simulink model "Schema_inteco_2"  (R2022b)
settings: Solver=VariableStepAuto  StartTime=0.0  StopTime=60  RelTol=1e-3
undefined symbols (not defined in the file): fm, g, Jm, Jphi, kb, kl, L, m, M, R, Ts, w
settings Model: Creator=Bogdana Cazan  LastModifiedBy=georg
settings SolverCC: AlgebraicLoopSolver=TrustRegion
settings DataIOCC: ReturnWorkspaceOutputs=off
settings DebuggingCC: UnconnectedInputMsg=warning  UnconnectedOutputMsg=warning  UnconnectedLineMsg=warning  SFMachineParentedDataDiag=warning  ArithmeticOperatorsInVariantConditions=warning
settings ModelReferenceCC: EnableRefExpFcnMdlSchedulingChecks=on
settings SFSimCC: CustomCodeUndefinedFunction=UseInterfaceOnly
settings RTWCC: DLArmComputeVersion=19.05

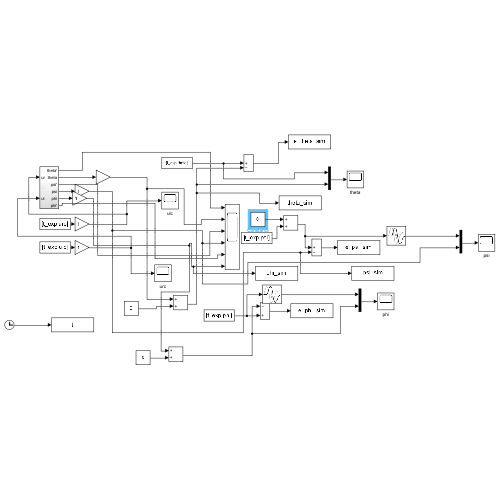
[thumbnail: Simulink's stored preview of the top-level diagram]
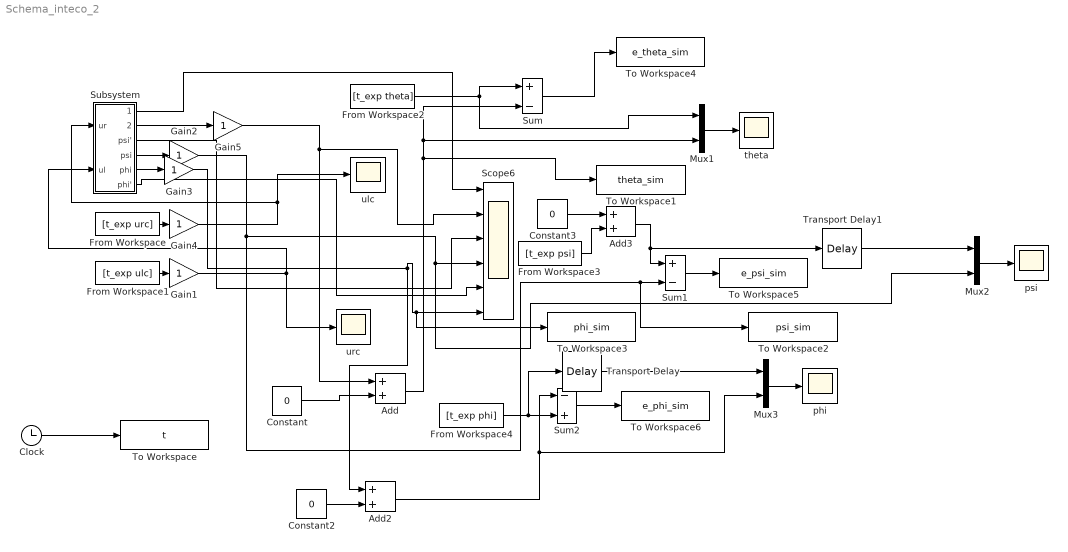
== system Schema_inteco_2 ==
  Add : Sum
  Add2 : Sum
  Add3 : Sum
  Clock : Clock
  Constant : Constant  Value=0
  Constant2 : Constant  Value=0
  Constant3 : Constant  Value=0
  From Workspace : FromWorkspace  VariableName=[t_exp urc]  SampleTime=Ts
  From Workspace1 : FromWorkspace  VariableName=[t_exp ulc]  SampleTime=Ts
  From Workspace2 : FromWorkspace  VariableName=[t_exp theta]  SampleTime=Ts
  From Workspace3 : FromWorkspace  VariableName=[t_exp psi]  SampleTime=Ts
  From Workspace4 : FromWorkspace  VariableName=[t_exp phi]  SampleTime=Ts
  Gain{1..5} (5 alike) : Gain
  Mux1 : Mux  Inputs=2
  Mux2 : Mux  Inputs=2
  Mux3 : Mux  Inputs=2
  Scope6 : Scope  NumInputPorts=6
  Subsystem : Subsystem
  Sum : Sum  Inputs=|+-
  Sum1 : Sum  Inputs=|+-
  Sum2 : Sum  Inputs=-+
  To Workspace : ToWorkspace  VariableName=t  SampleTime=Ts
  To Workspace1 : ToWorkspace  VariableName=theta_sim  SampleTime=Ts
  To Workspace2 : ToWorkspace  VariableName=psi_sim  SampleTime=Ts
  To Workspace3 : ToWorkspace  VariableName=phi_sim  SampleTime=Ts
  To Workspace4 : ToWorkspace  VariableName=e_theta_sim  SampleTime=Ts
  To Workspace5 : ToWorkspace  VariableName=e_psi_sim  SampleTime=Ts
  To Workspace6 : ToWorkspace  VariableName=e_phi_sim  SampleTime=Ts
  Transport Delay : TransportDelay  DelayTime=2.6
  Transport Delay1 : TransportDelay  DelayTime=1.2
  phi : Scope
  psi : Scope
  theta : Scope
  ulc : Scope
  urc : Scope
  wires:
  From Workspace/1 -> Gain4/1
  Subsystem/1(theta') -> Scope6/1
  Subsystem/3(psi') -> Scope6/3
  Subsystem/6(phi') -> Scope6/5
  Clock/1 -> To Workspace/1
  From Workspace2/1 -> Mux1/1, Sum/1
  Sum/1 -> To Workspace4/1
  From Workspace4/1 -> Transport Delay/1, Sum2/2
  Sum2/1 -> To Workspace6/1
  Mux1/1 -> theta/1
  Sum1/1 -> To Workspace5/1
  Mux2/1 -> psi/1
  Mux3/1 -> phi/1
  From Workspace1/1 -> Gain1/1
  Constant/1 -> Add/2
  Add/1 -> To Workspace1/1, Mux1/2, Sum/2
  Constant2/1 -> Add2/2
  Add2/1 -> Mux3/2, Sum2/1
  Gain1/1 -> Subsystem/2(ul), urc/1
  Gain4/1 -> ulc/1, Subsystem/1(ur)
  Subsystem/2(theta) -> Gain5/1
  Subsystem/4(psi) -> Gain2/1
  Subsystem/5(phi) -> Gain3/1
  Gain2/1 -> To Workspace2/1, Sum1/2, Mux2/2, Scope6/4
  Gain3/1 -> To Workspace3/1, Scope6/6, Add2/1
  Gain5/1 -> Add/1, Scope6/2
  Transport Delay/1 -> Mux3/1
  Add3/1 -> Transport Delay1/1, Sum1/1
  From Workspace3/1 -> Add3/2
  Constant3/1 -> Add3/1
  Transport Delay1/1 -> Mux2/1

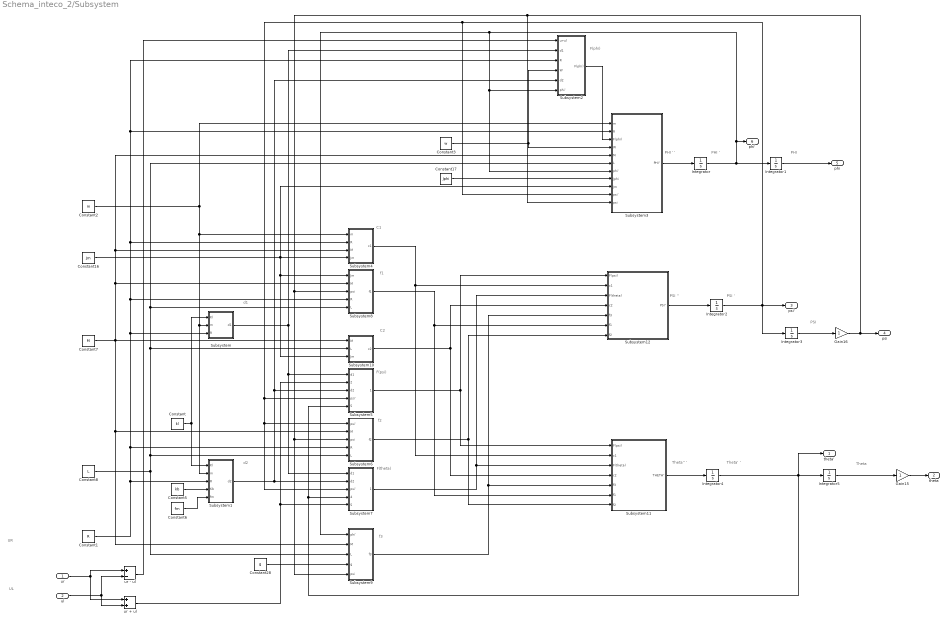
== system Schema_inteco_2/Subsystem ==
  note: f3
  note: d2
  note: F(psi)
  note: F(theta)
  note: f2
  note: Theta
  note: Theta' '
  note: Theta'' '
  note: PSI
  note: PSI '
  note: PSI ''
  note: f1
  note: C2
  note: UL
  note: UR
  note: C1
  note: PHI
  note: PHI '
  note: PHI ' '
  note: F(phi)
  note: d1
  ur : Inport
  ul : Inport  Port=2
  Constant : Constant  Value=kl
  Constant1 : Constant  Value=R
  Constant16 : Constant  Value=Jm
  Constant17 : Constant  Value=Jphi
  Constant2 : Constant  Value=m
  Constant28 : Constant  Value=g
  Constant3 : Constant  Value=w
  Constant5 : Constant  Value=kb
  Constant6 : Constant  Value=fm
  Constant7 : Constant  Value=M
  Constant8 : Constant  Value=L
  Gain15 : Gain
  Gain16 : Gain
  Integrator{,1..5} (6 alike) : Integrator
  Subsystem : Subsystem
  Subsystem1 : Subsystem
  Subsystem10 : Subsystem
  Subsystem11 : Subsystem
  Subsystem12 : Subsystem
  Subsystem2 : Subsystem
  Subsystem3 : Subsystem
  Subsystem4 : Subsystem
  Subsystem5 : Subsystem
  Subsystem6 : Subsystem
  Subsystem7 : Subsystem
  Subsystem8 : Subsystem
  Subsystem9 : Subsystem
  "ur + ul " : Sum
  ur - ul : Sum  Inputs=+-
  theta' : Outport  VectorParamsAs1DForOutWhenUnconnected=off
  theta : Outport  Port=2  VectorParamsAs1DForOutWhenUnconnected=off
  psi' : Outport  Port=3  VectorParamsAs1DForOutWhenUnconnected=off
  psi : Outport  Port=4  VectorParamsAs1DForOutWhenUnconnected=off
  phi : Outport  Port=5  VectorParamsAs1DForOutWhenUnconnected=off
  phi' : Outport  Port=6  VectorParamsAs1DForOutWhenUnconnected=off
  wires:
  Integrator3/1 -> Gain16/1
  ul/1 -> "ur + ul "/2, ur - ul/2
  Integrator2/1 -> Integrator3/1, Subsystem3/10(psi'), Subsystem6/1(psi'), Subsystem7/3(psi'), Subsystem5/4(psi'), psi'/1
  ur/1 -> "ur + ul "/1, ur - ul/1
  Constant2/1 -> Subsystem3/1(m), Subsystem4/1(m), Subsystem/2(m), Subsystem1/2(m)
  ur - ul/1 -> Subsystem2/1(ur-ul)
  Integrator4/1 -> Subsystem7/4(theta'), Subsystem5/5(theta'), Integrator5/1, theta'/1
  Constant6/1 -> Subsystem1/5(fm)
  Constant17/1 -> Subsystem3/8("Jphi ")
  Constant5/1 -> Subsystem1/4(Kb)
  Constant8/1 -> Subsystem9/3("L "), Subsystem10/2(L), Subsystem8/5(L), Subsystem3/6(L), Subsystem6/5(L)
  Constant/1 -> Subsystem/1(Kl), Subsystem1/1(Kl)
  Constant1/1 -> Subsystem3/2(R), Subsystem2/3(R), Subsystem4/2(R), Subsystem8/4("R "), Subsystem/3(R), Subsystem6/4(R), Subsystem1/3(R)
  Integrator1/1 -> phi/1
  Constant16/1 -> Subsystem3/9(Jm), Subsystem10/3(Jm), Subsystem8/1(Jm), Subsystem4/4(Jm)
  Subsystem/1(d1) -> Subsystem2/2(d1), Subsystem7/1(d1), Subsystem5/1(d1)
  Gain15/1 -> theta/1
  Subsystem6/1(f2) -> Subsystem12/7(f2), Subsystem11/7(f2)
  Constant7/1 -> Subsystem9/2(M), Subsystem6/2(M), Subsystem10/1(M), Subsystem3/5(M), Subsystem4/3(M), Subsystem8/2(M)
  Subsystem1/1(d2) -> Subsystem2/5(d2), Subsystem5/3(d2), Subsystem7/2(d2)
  "ur + ul "/1 -> Subsystem5/2(ur+ul), Subsystem7/5(ur+ul)
  Constant28/1 -> Subsystem9/4(g)
  Subsystem4/1(c1) -> Subsystem11/2(c1), Subsystem12/2(c1)
  Subsystem8/1(f1) -> Subsystem11/6(f1), Subsystem12/6(f1)
  Subsystem11/1("THETA\"") -> Integrator4/1
  Subsystem10/1(c2) -> Subsystem11/4(c2), Subsystem12/4(c2)
  Subsystem5/1(F(psi)) -> Subsystem11/1(F(psi)), Subsystem12/1(F(psi))
  Subsystem7/1(F(theta)) -> Subsystem12/3(F(theta)), Subsystem11/3(F(theta))
  Subsystem9/1(f3) -> Subsystem12/5(f3), Subsystem11/5(f3)
  Subsystem12/1("PSI\"") -> Integrator2/1
  Integrator5/1 -> Gain15/1
  Subsystem2/1(F(phi)) -> Subsystem3/3(F(phi))
  Gain16/1 -> Subsystem3/11(psi), Subsystem9/5(psi), Subsystem6/3(psi), Subsystem8/3(psi), psi/1
  Constant3/1 -> Subsystem2/4(W), Subsystem3/4(W)
  Subsystem3/1("PHI\"") -> Integrator/1
  Integrator/1 -> Subsystem3/7(phi'), Subsystem2/6(phi'), Subsystem9/1(phi'), phi'/1, Integrator1/1

== system Schema_inteco_2/Subsystem/Subsystem ==
  Kl : Inport
  m : Inport  Port=2
  R : Inport  Port=3
  Kl / (R*m) : Product  Inputs=*/
  R * m : Product
  d1 : Outport
  wires:
  m/1 -> R * m/2
  R/1 -> R * m/1
  Kl / (R*m)/1 -> d1/1
  Kl/1 -> Kl / (R*m)/1
  R * m/1 -> Kl / (R*m)/2

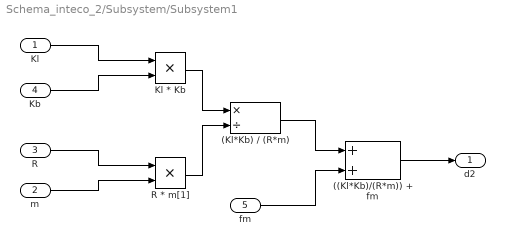
== system Schema_inteco_2/Subsystem/Subsystem1 ==
  Kl : Inport
  m : Inport  Port=2
  R : Inport  Port=3
  Kb : Inport  Port=4
  fm : Inport  Port=5
  ((Kl*Kb)/(R*m)) + fm : Sum
  (Kl*Kb) / (R*m) : Product  Inputs=*/
  Kl * Kb : Product
  R * m[1] : Product
  d2 : Outport
  wires:
  fm/1 -> ((Kl*Kb)/(R*m)) + fm/2
  Kl * Kb/1 -> (Kl*Kb) / (R*m)/1
  R/1 -> R * m[1]/1
  ((Kl*Kb)/(R*m)) + fm/1 -> d2/1
  (Kl*Kb) / (R*m)/1 -> ((Kl*Kb)/(R*m)) + fm/1
  m/1 -> R * m[1]/2
  R * m[1]/1 -> (Kl*Kb) / (R*m)/2
  Kb/1 -> Kl * Kb/2
  Kl/1 -> Kl * Kb/1

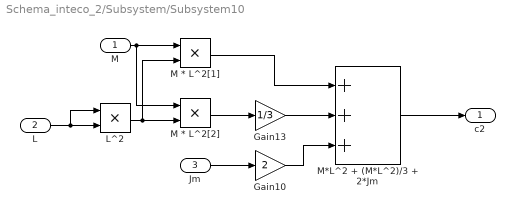
== system Schema_inteco_2/Subsystem/Subsystem10 ==
  M : Inport
  L : Inport  Port=2
  Jm : Inport  Port=3
  Gain10 : Gain  Gain=2
  Gain13 : Gain  Gain=1/3
  L^2 : Product
  M * L^2[1] : Product
  M * L^2[2] : Product
  M*L^2 + (M*L^2)/3 + 2*Jm : Sum  Inputs=+++
  c2 : Outport
  wires:
  L/1 -> L^2/1, L^2/2
  M/1 -> M * L^2[1]/1, M * L^2[2]/1
  Gain10/1 -> M*L^2 + (M*L^2)/3 + 2*Jm/3
  L^2/1 -> M * L^2[1]/2, M * L^2[2]/2
  Gain13/1 -> M*L^2 + (M*L^2)/3 + 2*Jm/2
  M * L^2[2]/1 -> Gain13/1
  M * L^2[1]/1 -> M*L^2 + (M*L^2)/3 + 2*Jm/1
  Jm/1 -> Gain10/1
  M*L^2 + (M*L^2)/3 + 2*Jm/1 -> c2/1

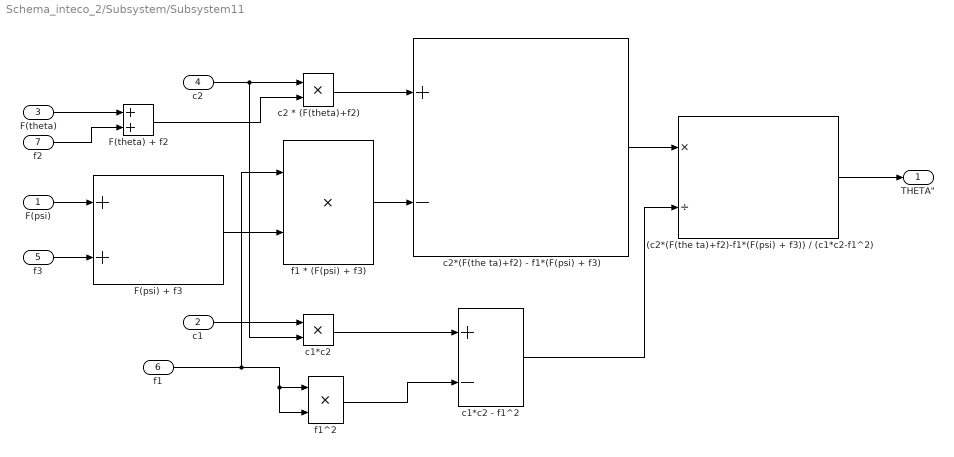
== system Schema_inteco_2/Subsystem/Subsystem11 ==
  F(psi) : Inport
  c1 : Inport  Port=2
  F(theta) : Inport  Port=3
  c2 : Inport  Port=4
  f3 : Inport  Port=5
  f1 : Inport  Port=6
  f2 : Inport  Port=7
  "  c1*c2 - f1^2" : Sum  Inputs=+-
  "(c2*(F(the ta)+f2)-f1*(F(psi) + f3)) / (c1*c2-f1^2) " : Product  Inputs=*/
  F(psi) + f3 : Sum
  F(theta) + f2 : Sum
  c1*c2 : Product
  c2 * (F(theta)+f2) : Product
  c2*(F(the ta)+f2) - f1*(F(psi) + f3) : Sum  Inputs=+-
  f1 * (F(psi) + f3) : Product
  f1^2 : Product
  "THETA\"" : Outport
  wires:
  f3/1 -> F(psi) + f3/2
  f1/1 -> f1^2/1, f1^2/2, f1 * (F(psi) + f3)/1
  F(theta)/1 -> F(theta) + f2/1
  c1/1 -> c1*c2/1
  f2/1 -> F(theta) + f2/2
  F(psi)/1 -> F(psi) + f3/1
  c2 * (F(theta)+f2)/1 -> c2*(F(the ta)+f2) - f1*(F(psi) + f3)/1
  F(psi) + f3/1 -> f1 * (F(psi) + f3)/2
  F(theta) + f2/1 -> c2 * (F(theta)+f2)/2
  c2/1 -> c1*c2/2, c2 * (F(theta)+f2)/1
  f1 * (F(psi) + f3)/1 -> c2*(F(the ta)+f2) - f1*(F(psi) + f3)/2
  c1*c2/1 -> "  c1*c2 - f1^2"/1
  f1^2/1 -> "  c1*c2 - f1^2"/2
  c2*(F(the ta)+f2) - f1*(F(psi) + f3)/1 -> "(c2*(F(the ta)+f2)-f1*(F(psi) + f3)) / (c1*c2-f1^2) "/1
  "  c1*c2 - f1^2"/1 -> "(c2*(F(the ta)+f2)-f1*(F(psi) + f3)) / (c1*c2-f1^2) "/2
  "(c2*(F(the ta)+f2)-f1*(F(psi) + f3)) / (c1*c2-f1^2) "/1 -> "THETA\""/1

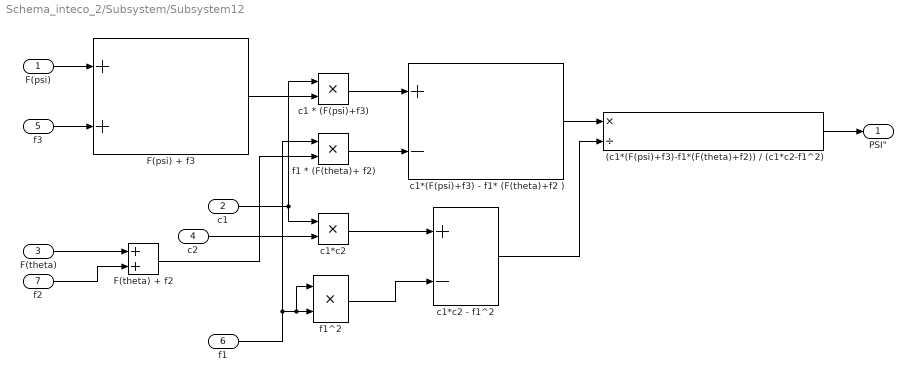
== system Schema_inteco_2/Subsystem/Subsystem12 ==
  F(psi) : Inport
  c1 : Inport  Port=2
  F(theta) : Inport  Port=3
  c2 : Inport  Port=4
  f3 : Inport  Port=5
  f1 : Inport  Port=6
  f2 : Inport  Port=7
  " c1*c2 - f1^2" : Sum  Inputs=+-
  (c1*(F(psi)+f3)-f1*(F(theta)+f2)) / (c1*c2-f1^2) : Product  Inputs=*/
  F(psi) + f3 : Sum
  F(theta) + f2 : Sum
  c1 * (F(psi)+f3) : Product
  c1*(F(psi)+f3) - f1* (F(theta)+f2 ) : Sum  Inputs=+-
  c1*c2 : Product
  f1 * (F(theta)+ f2) : Product
  f1^2 : Product
  "PSI\"" : Outport
  wires:
  f3/1 -> F(psi) + f3/2
  F(psi)/1 -> F(psi) + f3/1
  " c1*c2 - f1^2"/1 -> (c1*(F(psi)+f3)-f1*(F(theta)+f2)) / (c1*c2-f1^2)/2
  F(theta)/1 -> F(theta) + f2/1
  F(theta) + f2/1 -> f1 * (F(theta)+ f2)/2
  f2/1 -> F(theta) + f2/2
  F(psi) + f3/1 -> c1 * (F(psi)+f3)/2
  c1*c2/1 -> " c1*c2 - f1^2"/1
  c1/1 -> c1*c2/1, c1 * (F(psi)+f3)/1
  c2/1 -> c1*c2/2
  f1/1 -> f1^2/1, f1^2/2, f1 * (F(theta)+ f2)/1
  c1 * (F(psi)+f3)/1 -> c1*(F(psi)+f3) - f1* (F(theta)+f2 )/1
  f1 * (F(theta)+ f2)/1 -> c1*(F(psi)+f3) - f1* (F(theta)+f2 )/2
  f1^2/1 -> " c1*c2 - f1^2"/2
  c1*(F(psi)+f3) - f1* (F(theta)+f2 )/1 -> (c1*(F(psi)+f3)-f1*(F(theta)+f2)) / (c1*c2-f1^2)/1
  (c1*(F(psi)+f3)-f1*(F(theta)+f2)) / (c1*c2-f1^2)/1 -> "PSI\""/1

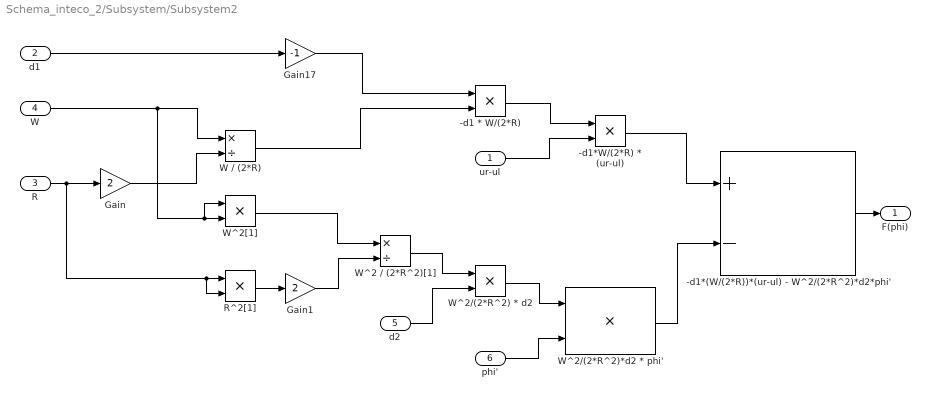
== system Schema_inteco_2/Subsystem/Subsystem2 ==
  ur-ul : Inport
  d1 : Inport  Port=2
  R : Inport  Port=3
  W : Inport  Port=4
  d2 : Inport  Port=5
  phi' : Inport  Port=6
  -d1 * W/(2*R) : Product
  -d1*(W/(2*R))*(ur-ul) - W^2/(2*R^2)*d2*phi' : Sum  Inputs=+-
  -d1*W/(2*R) * (ur-ul) : Product
  Gain : Gain  Gain=2
  Gain1 : Gain  Gain=2
  Gain17 : Gain  Gain=-1
  R^2[1] : Product
  W / (2*R) : Product  Inputs=*/
  W^2 / (2*R^2)[1] : Product  Inputs=*/
  W^2/(2*R^2) * d2 : Product
  W^2/(2*R^2)*d2 * phi' : Product
  W^2[1] : Product
  F(phi) : Outport
  wires:
  W^2/(2*R^2)*d2 * phi'/1 -> -d1*(W/(2*R))*(ur-ul) - W^2/(2*R^2)*d2*phi'/2
  R/1 -> Gain/1, R^2[1]/2, R^2[1]/1
  W^2[1]/1 -> W^2 / (2*R^2)[1]/1
  phi'/1 -> W^2/(2*R^2)*d2 * phi'/2
  -d1*W/(2*R) * (ur-ul)/1 -> -d1*(W/(2*R))*(ur-ul) - W^2/(2*R^2)*d2*phi'/1
  Gain/1 -> W / (2*R)/2
  W^2/(2*R^2) * d2/1 -> W^2/(2*R^2)*d2 * phi'/1
  W^2 / (2*R^2)[1]/1 -> W^2/(2*R^2) * d2/1
  W / (2*R)/1 -> -d1 * W/(2*R)/2
  R^2[1]/1 -> Gain1/1
  -d1*(W/(2*R))*(ur-ul) - W^2/(2*R^2)*d2*phi'/1 -> F(phi)/1
  Gain1/1 -> W^2 / (2*R^2)[1]/2
  -d1 * W/(2*R)/1 -> -d1*W/(2*R) * (ur-ul)/1
  d2/1 -> W^2/(2*R^2) * d2/2
  Gain17/1 -> -d1 * W/(2*R)/1
  ur-ul/1 -> -d1*W/(2*R) * (ur-ul)/2
  d1/1 -> Gain17/1
  W/1 -> W / (2*R)/1, W^2[1]/1, W^2[1]/2

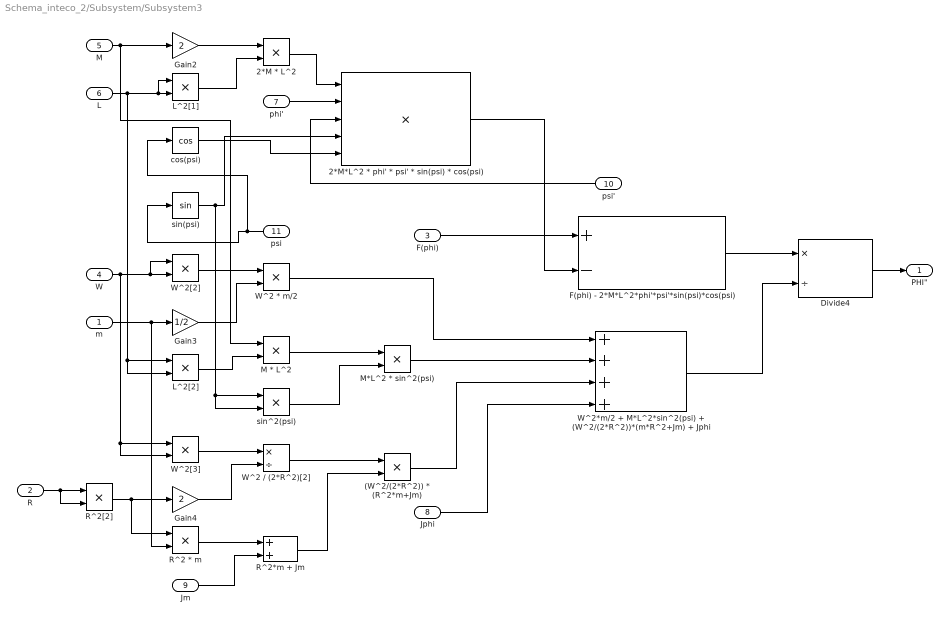
== system Schema_inteco_2/Subsystem/Subsystem3 ==
  m : Inport
  R : Inport  Port=2
  F(phi) : Inport  Port=3
  W : Inport  Port=4
  M : Inport  Port=5
  L : Inport  Port=6
  phi' : Inport  Port=7
  "Jphi " : Inport  Port=8
  Jm : Inport  Port=9
  psi' : Inport  Port=10
  psi : Inport  Port=11
  (W^2/(2*R^2)) * (R^2*m+Jm) : Product
  2*M * L^2 : Product
  2*M*L^2 * phi' * psi' * sin(psi) * cos(psi) : Product  Inputs=5
  Divide4 : Product  Inputs=*/
  F(phi) - 2*M*L^2*phi'*psi'*sin(psi)*cos(psi) : Sum  Inputs=+-
  Gain2 : Gain  Gain=2
  Gain3 : Gain  Gain=1/2
  Gain4 : Gain  Gain=2
  L^2[1] : Product
  L^2[2] : Product
  M * L^2 : Product
  M*L^2 * sin^2(psi) : Product
  R^2 * m : Product
  R^2*m + Jm : Sum
  R^2[2] : Product
  W^2 * m/2 : Product
  W^2 / (2*R^2)[2] : Product  Inputs=*/
  W^2*m/2 + M*L^2*sin^2(psi) + (W^2/(2*R^2))*(m*R^2+Jm) + Jphi : Sum  Inputs=++++
  W^2[2] : Product
  W^2[3] : Product
  cos(psi) : Trigonometry  Operator=cos
  sin(psi) : Trigonometry
  sin^2(psi) : Product
  "PHI\"" : Outport
  wires:
  m/1 -> Gain3/1, R^2 * m/2
  W/1 -> W^2[3]/1, W^2[3]/2, W^2[2]/1, W^2[2]/2
  W^2 / (2*R^2)[2]/1 -> (W^2/(2*R^2)) * (R^2*m+Jm)/1
  R/1 -> R^2[2]/2, R^2[2]/1
  psi'/1 -> 2*M*L^2 * phi' * psi' * sin(psi) * cos(psi)/3
  M/1 -> M * L^2/1, Gain2/1
  L/1 -> L^2[2]/2, L^2[2]/1, L^2[1]/1, L^2[1]/2
  W^2 * m/2/1 -> W^2*m/2 + M*L^2*sin^2(psi) + (W^2/(2*R^2))*(m*R^2+Jm) + Jphi/1
  L^2[1]/1 -> 2*M * L^2/2
  sin(psi)/1 -> sin^2(psi)/1, sin^2(psi)/2, 2*M*L^2 * phi' * psi' * sin(psi) * cos(psi)/4
  R^2[2]/1 -> R^2 * m/1, Gain4/1
  Gain2/1 -> 2*M * L^2/1
  cos(psi)/1 -> 2*M*L^2 * phi' * psi' * sin(psi) * cos(psi)/5
  W^2[2]/1 -> W^2 * m/2/1
  Gain3/1 -> W^2 * m/2/2
  L^2[2]/1 -> M * L^2/2
  W^2[3]/1 -> W^2 / (2*R^2)[2]/1
  Gain4/1 -> W^2 / (2*R^2)[2]/2
  R^2 * m/1 -> R^2*m + Jm/1
  Jm/1 -> R^2*m + Jm/2
  psi/1 -> cos(psi)/1, sin(psi)/1
  2*M * L^2/1 -> 2*M*L^2 * phi' * psi' * sin(psi) * cos(psi)/1
  phi'/1 -> 2*M*L^2 * phi' * psi' * sin(psi) * cos(psi)/2
  M * L^2/1 -> M*L^2 * sin^2(psi)/1
  F(phi) - 2*M*L^2*phi'*psi'*sin(psi)*cos(psi)/1 -> Divide4/1
  sin^2(psi)/1 -> M*L^2 * sin^2(psi)/2
  2*M*L^2 * phi' * psi' * sin(psi) * cos(psi)/1 -> F(phi) - 2*M*L^2*phi'*psi'*sin(psi)*cos(psi)/2
  R^2*m + Jm/1 -> (W^2/(2*R^2)) * (R^2*m+Jm)/2
  M*L^2 * sin^2(psi)/1 -> W^2*m/2 + M*L^2*sin^2(psi) + (W^2/(2*R^2))*(m*R^2+Jm) + Jphi/2
  F(phi)/1 -> F(phi) - 2*M*L^2*phi'*psi'*sin(psi)*cos(psi)/1
  (W^2/(2*R^2)) * (R^2*m+Jm)/1 -> W^2*m/2 + M*L^2*sin^2(psi) + (W^2/(2*R^2))*(m*R^2+Jm) + Jphi/3
  "Jphi "/1 -> W^2*m/2 + M*L^2*sin^2(psi) + (W^2/(2*R^2))*(m*R^2+Jm) + Jphi/4
  W^2*m/2 + M*L^2*sin^2(psi) + (W^2/(2*R^2))*(m*R^2+Jm) + Jphi/1 -> Divide4/2
  Divide4/1 -> "PHI\""/1

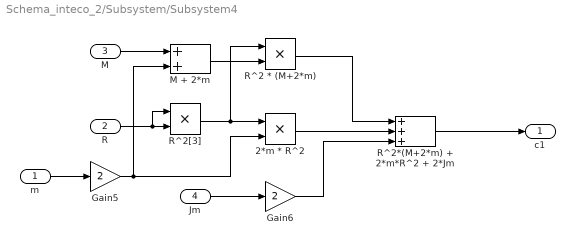
== system Schema_inteco_2/Subsystem/Subsystem4 ==
  m : Inport
  R : Inport  Port=2
  M : Inport  Port=3
  Jm : Inport  Port=4
  2*m * R^2 : Product
  Gain5 : Gain  Gain=2
  Gain6 : Gain  Gain=2
  M + 2*m : Sum
  R^2 * (M+2*m) : Product
  R^2*(M+2*m) + 2*m*R^2 + 2*Jm : Sum  Inputs=+++
  R^2[3] : Product
  c1 : Outport
  wires:
  m/1 -> Gain5/1
  R^2[3]/1 -> R^2 * (M+2*m)/1, 2*m * R^2/1
  M/1 -> M + 2*m/1
  R^2 * (M+2*m)/1 -> R^2*(M+2*m) + 2*m*R^2 + 2*Jm/1
  Jm/1 -> Gain6/1
  R/1 -> R^2[3]/1, R^2[3]/2
  Gain5/1 -> 2*m * R^2/2, M + 2*m/2
  M + 2*m/1 -> R^2 * (M+2*m)/2
  2*m * R^2/1 -> R^2*(M+2*m) + 2*m*R^2 + 2*Jm/2
  Gain6/1 -> R^2*(M+2*m) + 2*m*R^2 + 2*Jm/3
  R^2*(M+2*m) + 2*m*R^2 + 2*Jm/1 -> c1/1

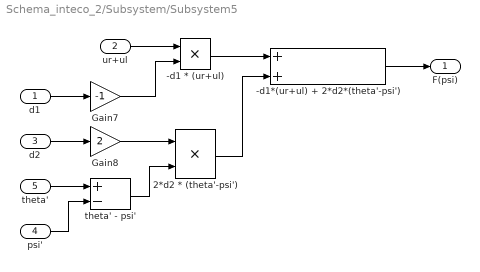
== system Schema_inteco_2/Subsystem/Subsystem5 ==
  d1 : Inport
  ur+ul : Inport  Port=2
  d2 : Inport  Port=3
  psi' : Inport  Port=4
  theta' : Inport  Port=5
  -d1 * (ur+ul) : Product
  -d1*(ur+ul) + 2*d2*(theta'-psi') : Sum
  2*d2 * (theta'-psi') : Product
  Gain7 : Gain  Gain=-1
  Gain8 : Gain  Gain=2
  theta' - psi' : Sum  Inputs=+-
  F(psi) : Outport
  wires:
  d1/1 -> Gain7/1
  ur+ul/1 -> -d1 * (ur+ul)/1
  psi'/1 -> theta' - psi'/2
  d2/1 -> Gain8/1
  theta' - psi'/1 -> 2*d2 * (theta'-psi')/2
  theta'/1 -> theta' - psi'/1
  Gain7/1 -> -d1 * (ur+ul)/2
  Gain8/1 -> 2*d2 * (theta'-psi')/1
  -d1 * (ur+ul)/1 -> -d1*(ur+ul) + 2*d2*(theta'-psi')/1
  2*d2 * (theta'-psi')/1 -> -d1*(ur+ul) + 2*d2*(theta'-psi')/2
  -d1*(ur+ul) + 2*d2*(theta'-psi')/1 -> F(psi)/1

== system Schema_inteco_2/Subsystem/Subsystem6 ==
  psi' : Inport
  M : Inport  Port=2
  psi : Inport  Port=3
  R : Inport  Port=4
  L : Inport  Port=5
  (psi')^2 : Product
  M * R * L * (psi')^2 * sin(psi) : Product  Inputs=5
  sin(psi) : Trigonometry
  f2 : Outport
  wires:
  L/1 -> M * R * L * (psi')^2 * sin(psi)/3
  psi/1 -> sin(psi)/1
  R/1 -> M * R * L * (psi')^2 * sin(psi)/2
  M/1 -> M * R * L * (psi')^2 * sin(psi)/1
  psi'/1 -> (psi')^2/2, (psi')^2/1
  sin(psi)/1 -> M * R * L * (psi')^2 * sin(psi)/4
  (psi')^2/1 -> M * R * L * (psi')^2 * sin(psi)/5
  M * R * L * (psi')^2 * sin(psi)/1 -> f2/1

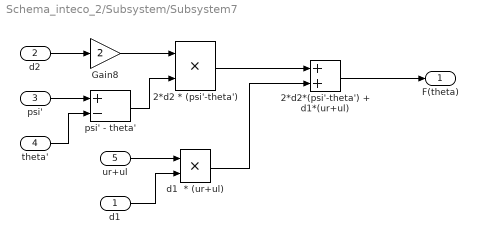
== system Schema_inteco_2/Subsystem/Subsystem7 ==
  d1 : Inport
  d2 : Inport  Port=2
  psi' : Inport  Port=3
  theta' : Inport  Port=4
  ur+ul : Inport  Port=5
  2*d2 * (psi'-theta') : Product
  "2*d2*(psi'-theta') + d1*(ur+ul) " : Sum
  Gain8 : Gain  Gain=2
  "d1  * (ur+ul) " : Product
  psi' - theta' : Sum  Inputs=+-
  F(theta) : Outport
  wires:
  ur+ul/1 -> "d1  * (ur+ul) "/1
  psi'/1 -> psi' - theta'/1
  d2/1 -> Gain8/1
  theta'/1 -> psi' - theta'/2
  Gain8/1 -> 2*d2 * (psi'-theta')/1
  psi' - theta'/1 -> 2*d2 * (psi'-theta')/2
  d1/1 -> "d1  * (ur+ul) "/2
  2*d2 * (psi'-theta')/1 -> "2*d2*(psi'-theta') + d1*(ur+ul) "/1
  "d1  * (ur+ul) "/1 -> "2*d2*(psi'-theta') + d1*(ur+ul) "/2
  "2*d2*(psi'-theta') + d1*(ur+ul) "/1 -> F(theta)/1

== system Schema_inteco_2/Subsystem/Subsystem8 ==
  Jm : Inport
  M : Inport  Port=2
  psi : Inport  Port=3
  "R " : Inport  Port=4
  L : Inport  Port=5
  Gain9 : Gain  Gain=2
  "M * R * L * cos(psi) " : Product  Inputs=4
  "M*R*L*cos(psi) - 2*Jm " : Sum  Inputs=+-
  cos(psi) : Trigonometry  Operator=cos
  f1 : Outport
  wires:
  cos(psi)/1 -> "M * R * L * cos(psi) "/4
  psi/1 -> cos(psi)/1
  "M*R*L*cos(psi) - 2*Jm "/1 -> f1/1
  L/1 -> "M * R * L * cos(psi) "/3
  M/1 -> "M * R * L * cos(psi) "/1
  Gain9/1 -> "M*R*L*cos(psi) - 2*Jm "/2
  "M * R * L * cos(psi) "/1 -> "M*R*L*cos(psi) - 2*Jm "/1
  "R "/1 -> "M * R * L * cos(psi) "/2
  Jm/1 -> Gain9/1

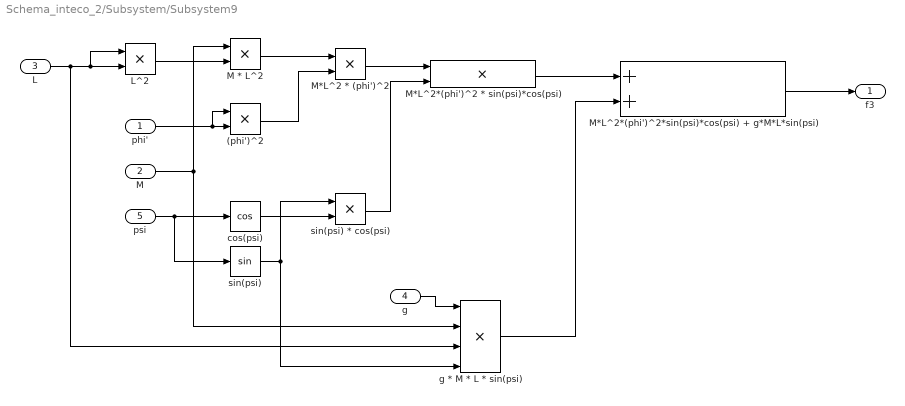
== system Schema_inteco_2/Subsystem/Subsystem9 ==
  phi' : Inport
  M : Inport  Port=2
  "L " : Inport  Port=3
  g : Inport  Port=4
  psi : Inport  Port=5
  (phi')^2 : Product
  L^2 : Product
  M * L^2 : Product
  M*L^2 * (phi')^2 : Product
  M*L^2*(phi')^2 * sin(psi)*cos(psi) : Product
  M*L^2*(phi')^2*sin(psi)*cos(psi) + g*M*L*sin(psi) : Sum
  cos(psi) : Trigonometry  Operator=cos
  g * M * L * sin(psi) : Product  Inputs=4
  sin(psi) : Trigonometry
  sin(psi) * cos(psi) : Product
  f3 : Outport
  wires:
  "L "/1 -> L^2/1, L^2/2, g * M * L * sin(psi)/3
  (phi')^2/1 -> M*L^2 * (phi')^2/2
  L^2/1 -> M * L^2/2
  phi'/1 -> (phi')^2/1, (phi')^2/2
  M/1 -> g * M * L * sin(psi)/2, M * L^2/1
  M * L^2/1 -> M*L^2 * (phi')^2/1
  psi/1 -> cos(psi)/1, sin(psi)/1
  cos(psi)/1 -> sin(psi) * cos(psi)/2
  g/1 -> g * M * L * sin(psi)/1
  sin(psi)/1 -> g * M * L * sin(psi)/4, sin(psi) * cos(psi)/1
  M*L^2 * (phi')^2/1 -> M*L^2*(phi')^2 * sin(psi)*cos(psi)/1
  sin(psi) * cos(psi)/1 -> M*L^2*(phi')^2 * sin(psi)*cos(psi)/2
  g * M * L * sin(psi)/1 -> M*L^2*(phi')^2*sin(psi)*cos(psi) + g*M*L*sin(psi)/2
  M*L^2*(phi')^2 * sin(psi)*cos(psi)/1 -> M*L^2*(phi')^2*sin(psi)*cos(psi) + g*M*L*sin(psi)/1
  M*L^2*(phi')^2*sin(psi)*cos(psi) + g*M*L*sin(psi)/1 -> f3/1
